simulink model "idealMode_pid_feedback_frontback"  (R2016b)
settings: Solver=ode15s  StartTime=0.0  StopTime=0.3  RelTol=1e-3
libraries: simulink x11
settings Model: Creator=chenb  LastModifiedBy=chenb

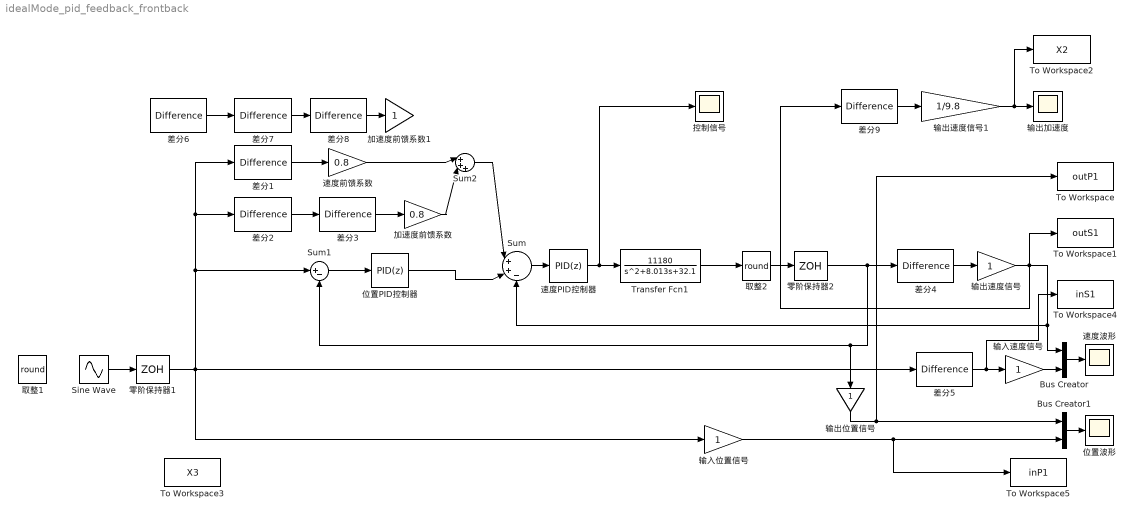
== system idealMode_pid_feedback_frontback ==
  Bus Creator : BusCreator  Inputs=2
  Bus Creator1 : BusCreator  Inputs=2
  Sine Wave : Sin  Amplitude=2000  Frequency=62.8  SampleTime=0
  Sum : Sum  Inputs=|++-
  Sum1 : Sum  Inputs=|+-
  Sum2 : Sum  Inputs=|+++
  To Workspace : ToWorkspace  VariableName=outP1  SampleTime=0.00025
      settings: Save2DSignal=2-D array (concatenate along first dimension)
  To Workspace1 : ToWorkspace  VariableName=outS1  SampleTime=0.00025
      settings: Save2DSignal=2-D array (concatenate along first dimension)
  To Workspace2 : ToWorkspace  VariableName=X2  SampleTime=0.00025
      settings: Save2DSignal=2-D array (concatenate along first dimension)
  To Workspace3 : ToWorkspace  VariableName=X3  SampleTime=0.00025
      settings: Save2DSignal=2-D array (concatenate along first dimension)
  To Workspace4 : ToWorkspace  VariableName=inS1  SampleTime=0.00025
      settings: Save2DSignal=2-D array (concatenate along first dimension)
  To Workspace5 : ToWorkspace  VariableName=inP1  SampleTime=0.00025
      settings: Save2DSignal=2-D array (concatenate along first dimension)
  Transfer Fcn1 : TransferFcn  Numerator=[11180]  Denominator=[1 8.013 32.1]
  位置PID控制器 : simulink/Continuous/PID Controller  Controller=PID  TimeDomain=Discrete-time  SampleTime=0.00025  IntegratorMethod=Forward Euler  FilterMethod=Forward Euler  Form=Parallel  UseFilter=on  ControllerParametersSource=internal  P=1  I=100  D=0  N=100  InitialConditionSource=internal  InitialConditionForIntegrator=0  InitialConditionForFilter=0  ExternalReset=none  LimitOutput=off  UpperSaturationLimit=inf  LowerSaturationLimit=-inf  LinearizeAsGain=on  AntiWindupMode=none  Kb=1  TrackingMode=off  Kt=1  PParamMin=[]  PParamMax=[]  IParamMin=[]  IParamMax=[]  DParamMin=[]  DParamMax=[]  NParamMin=[]  NParamMax=[]  KbParamMin=[]  KbParamMax=[]  KtParamMin=[]  KtParamMax=[]  POutMin=[]  POutMax=[]  IOutMin=[]  IOutMax=[]  DOutMin=[]  DOutMax=[]  NOutMin=[]  NOutMax=[]  KbOutMin=[]  KbOutMax=[]  KtOutMin=[]  KtOutMax=[]  IntegratorOutMin=[]  IntegratorOutMax=[]  FilterOutMin=[]  FilterOutMax=[]  SumOutMin=[]  SumOutMax=[]  SumI1OutMin=[]  SumI1OutMax=[]  SumI2OutMin=[]  SumI2OutMax=[]  SumI3OutMin=[]  SumI3OutMax=[]  SumDOutMin=[]  SumDOutMax=[]  SaturationOutMin=[]  SaturationOutMax=[]  IntegratorContinuousStateAttributes=''  IntegratorStateMustResolveToSignalObject=off  IntegratorRTWStateStorageClass=Auto  FilterContinuousStateAttributes=''  FilterStateMustResolveToSignalObject=off  FilterRTWStateStorageClass=Auto  DifferentiatorICPrevScaledInput=0  DifferentiatorOutMin=[]  DifferentiatorOutMax=[]
  位置波形 : Scope
  加速度前馈系数 : Gain  Gain=0.8
  加速度前馈系数1 : Gain
  取整1 : Rounding  Operator=round
  取整2 : Rounding  Operator=round
  差分{1..9} (9 alike) : simulink/Discrete/Difference  ICPrevInput=0.0  OutMin=[]  OutMax=[]  OutDataType=fixdt(1, 16)  OutScaling=2^-10  DoSatur=off
  控制信号 : Scope
  输入位置信号 : Gain
  输入速度信号 : Gain
  输出位置信号 : Gain
  输出加速度 : Scope
  输出速度信号 : Gain
  输出速度信号1 : Gain  Gain=1/9.8
  速度PID控制器 : simulink/Continuous/PID Controller  Controller=PID  TimeDomain=Discrete-time  SampleTime=0.00025  IntegratorMethod=Forward Euler  FilterMethod=Forward Euler  Form=Parallel  UseFilter=on  ControllerParametersSource=internal  P=700  I=500  D=0  N=100  InitialConditionSource=internal  InitialConditionForIntegrator=0  InitialConditionForFilter=0  ExternalReset=none  LimitOutput=off  UpperSaturationLimit=inf  LowerSaturationLimit=-inf  LinearizeAsGain=on  AntiWindupMode=none  Kb=1  TrackingMode=off  Kt=1  PParamMin=[]  PParamMax=[]  IParamMin=[]  IParamMax=[]  DParamMin=[]  DParamMax=[]  NParamMin=[]  NParamMax=[]  KbParamMin=[]  KbParamMax=[]  KtParamMin=[]  KtParamMax=[]  POutMin=[]  POutMax=[]  IOutMin=[]  IOutMax=[]  DOutMin=[]  DOutMax=[]  NOutMin=[]  NOutMax=[]  KbOutMin=[]  KbOutMax=[]  KtOutMin=[]  KtOutMax=[]  IntegratorOutMin=[]  IntegratorOutMax=[]  FilterOutMin=[]  FilterOutMax=[]  SumOutMin=[]  SumOutMax=[]  SumI1OutMin=[]  SumI1OutMax=[]  SumI2OutMin=[]  SumI2OutMax=[]  SumI3OutMin=[]  SumI3OutMax=[]  SumDOutMin=[]  SumDOutMax=[]  SaturationOutMin=[]  SaturationOutMax=[]  IntegratorContinuousStateAttributes=''  IntegratorStateMustResolveToSignalObject=off  IntegratorRTWStateStorageClass=Auto  FilterContinuousStateAttributes=''  FilterStateMustResolveToSignalObject=off  FilterRTWStateStorageClass=Auto  DifferentiatorICPrevScaledInput=0  DifferentiatorOutMin=[]  DifferentiatorOutMax=[]
  速度前馈系数 : Gain  Gain=0.8
  速度波形 : Scope
  零阶保持器1 : ZeroOrderHold  SampleTime=0.00025
  零阶保持器2 : ZeroOrderHold  SampleTime=0.00025
  wires:
  零阶保持器1/1 -> 输入位置信号/1, 差分5/1, 差分1/1, 差分2/1, Sum1/1
  Bus Creator/1 -> 速度波形/1
  Sum/1 -> 速度PID控制器/1
  差分4/1 -> 输出速度信号/1
  输出速度信号/1 -> 差分9/1, To Workspace1/1, Sum/3, Bus Creator/1
  速度PID控制器/1 -> 控制信号/1, Transfer Fcn1/1
  Bus Creator1/1 -> 位置波形/1
  ? -> 取整1/1, To Workspace3/1
  差分5/1 -> To Workspace4/1, 输入速度信号/1
  取整2/1 -> 零阶保持器2/1
  Sum1/1 -> 位置PID控制器/1
  零阶保持器2/1 -> Sum1/2, 输出位置信号/1, 差分4/1
  差分2/1 -> 差分3/1
  差分1/1 -> 速度前馈系数/1
  差分3/1 -> 加速度前馈系数/1
  位置PID控制器/1 -> Sum/2
  加速度前馈系数/1 -> Sum2/2
  速度前馈系数/1 -> Sum2/1
  Sum2/1 -> Sum/1
  输入位置信号/1 -> To Workspace5/1, Bus Creator1/2
  输入速度信号/1 -> Bus Creator/2
  输出位置信号/1 -> To Workspace/1, Bus Creator1/1
  Transfer Fcn1/1 -> 取整2/1
  差分6/1 -> 差分7/1
  差分7/1 -> 差分8/1
  差分8/1 -> 加速度前馈系数1/1
  差分9/1 -> 输出速度信号1/1
  输出速度信号1/1 -> To Workspace2/1, 输出加速度/1
  Sine Wave/1 -> 零阶保持器1/1
